simulink library "inp"  (R2021b)
settings: Solver=VariableStepAuto  StartTime=0.0  StopTime=10.0  RelTol=1e-3
undefined symbols (not defined in the file): C_TASK_5MS_S, FALSE, KINP_AcoreReadyToSlp_flg_ovrdflg, KINP_AcoreReadyToSlp_flg_ovrdval, KINP_AllowMovThd_OTA_enum_ovrdflg, KINP_AllowMovThd_OTA_enum_ovrdval, KINP_APSAngleTarget_Deg_ovrdflg, KINP_APSAngleTarget_Deg_ovrdval, KINP_APSDecReq_mps2_ovrdflg, KINP_APSDecReq_mps2_ovrdval, KINP_APSDecReqA_flg_ovrdflg, KINP_APSDecReqA_flg_ovrdval, KINP_APSDFLL_cm_ovrdflg, KINP_APSDFLL_cm_ovrdval, KINP_APSDFLR_cm_ovrdflg, KINP_APSDFLR_cm_ovrdval, KINP_APSDRLL_cm_ovrdflg, KINP_APSDRLL_cm_ovrdval, KINP_APSDRLR_cm_ovrdflg, KINP_APSDRLR_cm_ovrdval, KINP_APSExitCondition_enum_ovrdflg, KINP_APSExitCondition_enum_ovrdval, KINP_APSHWVer_enum_ovrdflg, KINP_APSHWVer_enum_ovrdval, KINP_APSProgressPCT_pct_ovrdflg, KINP_APSProgressPCT_pct_ovrdval, KINP_APSPwrReq_enum_ovrdflg, KINP_APSPwrReq_enum_ovrdval, KINP_APSReq_enum_ovrdflg, KINP_APSReq_enum_ovrdval, KINP_APSRQDisplay_enum_ovrdflg, KINP_APSRQDisplay_enum_ovrdval, KINP_APSRqEPASCtrl_flg_ovrdflg, KINP_APSRqEPASCtrl_flg_ovrdval, KINP_APSShiftPosnReq_enum_ovrdval, KINP_APSShiftPosnReq_enum_ovrflg, KINP_APSSpeedCMD_kph_ovrdval, KINP_APSSpeedCMD_kph_ovrflg, KINP_APSStaSystem_enum_ovrdflg, KINP_APSStaSystem_enum_ovrdval, KINP_APSSWVer_enum_ovrdflg, KINP_APSSWVer_enum_ovrdval, KINP_APSVMCReqA_flg_ovrdval, KINP_APSVMCReqA_flg_ovrflg, KINP_APSVRqEPASCtrl_flg_ovrdflg, KINP_APSVRqEPASCtrl_flg_ovrdval, KINP_AuxBattVolmV_mV_ovrdflg, KINP_AuxBattVolmV_mV_ovrdval, KINP_CAASSta_enum_ovrdflg, KINP_CAASSta_enum_ovrdval, KINP_CAASVMCReqA_flg_ovrdval, KINP_CAASVMCReqA_flg_ovrflg, KINP_CAN1BusOff_flg_ovrdflg, KINP_CAN1BusOff_flg_ovrdval, KINP_CAN2BusOff_flg_ovrdflg, KINP_CAN2BusOff_flg_ovrdval, KINP_CAN3BusOff_flg_ovrdflg, KINP_CAN3BusOff_flg_ovrdval, KINP_CAN4BusOff_flg_ovrdflg, KINP_CAN4BusOff_flg_ovrdval ... (+152)
libraries: FVT_lib x1035, hcu_lib x1
(part 3 of 33)

== system inp/INP/TPMS ==
  BHAL_TPMS_outputs : Inport  OutDataTypeStr=Bus: BHAL_TPMS_outputs
  Bus Creator : BusCreator  Inputs=52  OutDataTypeStr=Bus: BINP_TPMS_outputs  NonVirtualBus=on
  Bus Selector : BusSelector  OutputSignals=VHAL_TPMSDataIn_flg,VHAL_TPMSID_raw,VHAL_TPMSPressure_raw,VHAL_TPMSTemp_raw,VHAL_TPMSSta_enum,VHAL_TPMSPressureMi_raw,VHAL_TPMSCRC_crc,VHAL_TPMSCRCCalc_crc,VHAL_TPMSFAT_flg,VHAL_TPMSBattLow_flg,VHAL_TPMSStorge_flg,VHAL_LFID_raw,VHAL_RFID_raw,VHAL_LRID_raw,VHAL_RRID_raw,VHAL_ChkStorge_flg,VHAL_ChkLFID_raw,VHAL_ChkRFID_raw,VHAL_ChkLRID_raw,VHAL_ChkRRID_raw,VHAL_FlashLFSensorFail_flg,VHAL_FlashRFSensorFail_flg,VHAL_FlashLRSensorFail_flg,VHAL_FlashRRSensorFail_flg,VHAL_FlashLFWheelPSW_raw8,VHAL_FlashRFWheelPSW_raw8,VHAL_FlashLRWheelPSW_raw8,VHAL_FlashRRWheelPSW_raw8,VHAL_FlashLFPindi_enum,VHAL_FlashRFPindi_enum,VHAL_FlashLRPindi_enum,VHAL_FlashRRPindi_enum,VHAL_FlashLFP20_raw8,VHAL_FlashRFP20_raw8,VHAL_FlashLRP20_raw8,VHAL_FlashRRP20_raw8,VHAL_FlashLFWheelPress_raw8,VHAL_FlashRFWheelPress_raw8,VHAL_FlashLRWheelPress_raw8,VHAL_FlashRRWheelPress_raw8,VHAL_FlashLFWheelTemp_C,VHAL_FlashRFWheelTemp_C,VHAL_FlashLRWheelTemp_C,VHAL_FlashRRWheelTemp_C,VHAL_FlashunlearnSfali_flg,VHAL_S1ID_raw,VHAL_S2ID_raw,VHAL_S3ID_raw,VHAL_S4ID_raw,VHAL_Prepresstemptrust_flg,VHAL_TPMSSensorIDRegSta_enum,VHAL_TPMSTrigger_flg
  Data Type Conversion{,8..10,15,26,28,45..48,55} (12 alike) : DataTypeConversion  OutDataTypeStr=boolean
  Data Type Conversion{1,11..14,16..19,22..25} (13 alike) : DataTypeConversion  OutDataTypeStr=uint32
  Data Type Conversion{2..7,20..21,27,32,34..35,37..44,49..54,56} (27 alike) : DataTypeConversion  OutDataTypeStr=uint8
  Subsystem : Subsystem
  Subsystem1 : Subsystem
  Subsystem10 : Subsystem
  Subsystem11 : Subsystem
  Subsystem12 : Subsystem
  Subsystem13 : Subsystem
  Subsystem14 : Subsystem
  Subsystem2 : Subsystem
  Subsystem3 : Subsystem
  Subsystem4 : Subsystem
  Subsystem5 : Subsystem
  Subsystem6 : Subsystem
  Subsystem7 : Subsystem
  Subsystem8 : Subsystem
  Subsystem9 : Subsystem
  BINP_TPMS_outputs : Outport  OutDataTypeStr=Bus: BINP_TPMS_outputs
  wires:
  Bus Selector/49 -> Data Type Conversion25/1  "<VHAL_S4ID_raw>"
  Bus Selector/48 -> Data Type Conversion24/1  "<VHAL_S3ID_raw>"
  Bus Selector/47 -> Data Type Conversion23/1  "<VHAL_S2ID_raw>"
  Bus Selector/46 -> Data Type Conversion22/1  "<VHAL_S1ID_raw>"
  Data Type Conversion25/1 -> Bus Creator/49  "VINP_S4ID_raw"
  Data Type Conversion24/1 -> Bus Creator/48  "VINP_S3ID_raw"
  Data Type Conversion23/1 -> Bus Creator/47  "VINP_S2ID_raw"
  Data Type Conversion22/1 -> Bus Creator/46  "VINP_S1ID_raw"
  Data Type Conversion21/1 -> Bus Creator/44  "VINP_FlashRRWheelTemp_C"
  Data Type Conversion20/1 -> Bus Creator/43  "VINP_FlashLRWheelTemp_C"
  Bus Selector/44 -> Data Type Conversion21/1  "<VHAL_FlashRRWheelTemp_C>"
  Bus Selector/43 -> Data Type Conversion20/1  "<VHAL_FlashLRWheelTemp_C>"
  Data Type Conversion55/1 -> Bus Creator/45  "VINP_FlashunlearnSfali_flg"
  Bus Selector/45 -> Data Type Conversion55/1  "<VHAL_FlashunlearnSfali_flg>"
  Data Type Conversion44/1 -> Bus Creator/42  "VINP_FlashRFWheelTemp_C"
  Bus Selector/42 -> Data Type Conversion44/1  "<VHAL_FlashRFWheelTemp_C>"
  Data Type Conversion43/1 -> Bus Creator/41  "VINP_FlashLFWheelTemp_C"
  Bus Selector/41 -> Data Type Conversion43/1  "<VHAL_FlashLFWheelTemp_C>"
  Data Type Conversion54/1 -> Bus Creator/40  "VINP_FlashRRWheelPress_raw8"
  Data Type Conversion42/1 -> Bus Creator/39  "VINP_FlashLRWheelPress_raw8"
  Bus Selector/40 -> Data Type Conversion54/1  "<VHAL_FlashRRWheelPress_raw8>"
  Bus Selector/39 -> Data Type Conversion42/1  "<VHAL_FlashLRWheelPress_raw8>"
  Data Type Conversion34/1 -> Bus Creator/38  "VINP_FlashRFWheelPress_raw8"
  Bus Selector/38 -> Data Type Conversion34/1  "<VHAL_FlashRFWheelPress_raw8>"
  Data Type Conversion56/1 -> Bus Creator/37  "VINP_FlashLFWheelPress_raw8"
  Bus Selector/37 -> Data Type Conversion56/1  "<VHAL_FlashLFWheelPress_raw8>"
  Data Type Conversion41/1 -> Bus Creator/36  "VINP_FlashRRP20_raw8"
  Bus Selector/36 -> Data Type Conversion41/1  "<VHAL_FlashRRP20_raw8>"
  Data Type Conversion39/1 -> Bus Creator/35  "VINP_FlashLRP20_raw8"
  Bus Selector/35 -> Data Type Conversion39/1  "<VHAL_FlashLRP20_raw8>"
  Data Type Conversion38/1 -> Bus Creator/34  "VINP_FlashRFP20_raw8"
  Bus Selector/34 -> Data Type Conversion38/1  "<VHAL_FlashRFP20_raw8>"
  Data Type Conversion40/1 -> Bus Creator/33  "VINP_FlashLFP20_raw8"
  Bus Selector/33 -> Data Type Conversion40/1  "<VHAL_FlashLFP20_raw8>"
  Data Type Conversion37/1 -> Bus Creator/32  "VINP_FlashRRPindi_enum"
  Bus Selector/32 -> Data Type Conversion37/1  "<VHAL_FlashRRPindi_enum>"
  Data Type Conversion35/1 -> Bus Creator/31  "VINP_FlashLRPindi_enum"
  Bus Selector/31 -> Data Type Conversion35/1  "<VHAL_FlashLRPindi_enum>"
  Data Type Conversion53/1 -> Bus Creator/30  "VINP_FlashRFPindi_enum"
  Bus Selector/30 -> Data Type Conversion53/1  "<VHAL_FlashRFPindi_enum>"
  Data Type Conversion32/1 -> Bus Creator/29  "VINP_FlashLFPindi_enum"
  Bus Selector/29 -> Data Type Conversion32/1  "<VHAL_FlashLFPindi_enum>"
  Data Type Conversion52/1 -> Bus Creator/28  "VINP_FlashRRWheelPSW_raw8"
  Bus Selector/28 -> Data Type Conversion52/1  "<VHAL_FlashRRWheelPSW_raw8>"
  Data Type Conversion50/1 -> Bus Creator/27  "VINP_FlashLRWheelPSW_raw8"
  Bus Selector/27 -> Data Type Conversion50/1  "<VHAL_FlashLRWheelPSW_raw8>"
  Data Type Conversion49/1 -> Bus Creator/26  "VINP_FlashRFWheelPSW_raw8"
  Bus Selector/26 -> Data Type Conversion49/1  "<VHAL_FlashRFWheelPSW_raw8>"
  Data Type Conversion51/1 -> Bus Creator/25  "VINP_FlashLFWheelPSW_raw8"
  Bus Selector/25 -> Data Type Conversion51/1  "<VHAL_FlashLFWheelPSW_raw8>"
  Data Type Conversion48/1 -> Bus Creator/24  "VINP_FlashRRSensorFail_flg"
  Bus Selector/24 -> Data Type Conversion48/1  "<VHAL_FlashRRSensorFail_flg>"
  Data Type Conversion47/1 -> Bus Creator/23  "VINP_FlashLRSensorFail_flg"
  Bus Selector/23 -> Data Type Conversion47/1  "<VHAL_FlashLRSensorFail_flg>"
  Data Type Conversion46/1 -> Bus Creator/22  "VINP_FlashRFSensorFail_flg"
  Bus Selector/22 -> Data Type Conversion46/1  "<VHAL_FlashRFSensorFail_flg>"
  Data Type Conversion45/1 -> Bus Creator/21  "VINP_FlashLFSensorFail_flg"
  Bus Selector/21 -> Data Type Conversion45/1  "<VHAL_FlashLFSensorFail_flg>"
  Data Type Conversion19/1 -> Bus Creator/20  "VINP_ChkRRID_raw"
  Data Type Conversion18/1 -> Bus Creator/19  "VINP_ChkLRID_raw"
  Data Type Conversion17/1 -> Bus Creator/18  "VINP_ChkRFID_raw"
  Data Type Conversion16/1 -> Bus Creator/17  "VINP_ChkLFID_raw"
  Data Type Conversion15/1 -> Bus Creator/16  "VINP_ChkStorge_flg"
  Bus Selector/20 -> Data Type Conversion19/1  "<VHAL_ChkRRID_raw>"
  Bus Selector/19 -> Data Type Conversion18/1  "<VHAL_ChkLRID_raw>"
  Bus Selector/18 -> Data Type Conversion17/1  "<VHAL_ChkRFID_raw>"
  Bus Selector/17 -> Data Type Conversion16/1  "<VHAL_ChkLFID_raw>"
  Bus Selector/16 -> Data Type Conversion15/1  "<VHAL_ChkStorge_flg>"
  Data Type Conversion14/1 -> Bus Creator/15  "VINP_RRID_raw"
  Data Type Conversion13/1 -> Bus Creator/14  "VINP_LRID_raw"
  Data Type Conversion12/1 -> Bus Creator/13  "VINP_RFID_raw"
  Data Type Conversion11/1 -> Bus Creator/12  "VINP_LFID_raw"
  Subsystem14/1(Out1) -> Data Type Conversion14/1
  Subsystem13/1(Out1) -> Data Type Conversion13/1
  Subsystem12/1(Out1) -> Data Type Conversion12/1
  Subsystem11/1(Out1) -> Data Type Conversion11/1
  Bus Selector/15 -> Subsystem14/1(In1)  "<VHAL_RRID_raw>"
  Bus Selector/14 -> Subsystem13/1(In1)  "<VHAL_LRID_raw>"
  Bus Selector/13 -> Subsystem12/1(In1)  "<VHAL_RFID_raw>"
  Bus Selector/12 -> Subsystem11/1(In1)  "<VHAL_LFID_raw>"
  Data Type Conversion10/1 -> Bus Creator/11  "VINP_TPMSStorge_flg"
  Subsystem10/1(Out1) -> Data Type Conversion10/1
  Bus Selector/11 -> Subsystem10/1(In1)  "<VHAL_TPMSStorge_flg>"
  Subsystem9/1(Out1) -> Data Type Conversion9/1
  Subsystem8/1(Out1) -> Data Type Conversion8/1
  Bus Selector/10 -> Subsystem9/1(In1)  "<VHAL_TPMSBattLow_flg>"
  Bus Selector/9 -> Subsystem8/1(In1)  "<VHAL_TPMSFAT_flg>"
  Data Type Conversion9/1 -> Bus Creator/10  "VINP_TPMSBattLow_flg"
  Data Type Conversion8/1 -> Bus Creator/9  "VINP_TPMSFAT_flg"
  Bus Creator/1 -> BINP_TPMS_outputs/1
  Data Type Conversion7/1 -> Bus Creator/8  "VINP_TPMSCRCCalc_crc"
  Data Type Conversion6/1 -> Bus Creator/7  "VINP_TPMSCRC_crc"
  Data Type Conversion5/1 -> Bus Creator/6  "VINP_TPMSPressureMi_raw"
  Data Type Conversion4/1 -> Bus Creator/5  "VINP_TPMSSta_enum"
  Data Type Conversion3/1 -> Bus Creator/4  "VINP_TPMSTemp_raw"
  Data Type Conversion2/1 -> Bus Creator/3  "VINP_TPMSPressure_raw"
  Data Type Conversion1/1 -> Bus Creator/2  "VINP_TPMSID_raw"
  Data Type Conversion/1 -> Bus Creator/1  "VINP_TPMSDataIn_flg"
  Subsystem7/1(Out1) -> Data Type Conversion7/1
  Subsystem6/1(Out1) -> Data Type Conversion6/1
  Subsystem5/1(Out1) -> Data Type Conversion5/1
  Subsystem4/1(Out1) -> Data Type Conversion4/1
  Subsystem3/1(Out1) -> Data Type Conversion3/1
  Subsystem2/1(Out1) -> Data Type Conversion2/1
  Subsystem1/1(Out1) -> Data Type Conversion1/1
  Subsystem/1(Out1) -> Data Type Conversion/1
  Bus Selector/8 -> Subsystem7/1(In1)  "<VHAL_TPMSCRCCalc_crc>"
  Bus Selector/7 -> Subsystem6/1(In1)  "<VHAL_TPMSCRC_crc>"
  Bus Selector/6 -> Subsystem5/1(In1)  "<VHAL_TPMSPressureMi_raw>"
  Bus Selector/5 -> Subsystem4/1(In1)  "<VHAL_TPMSSta_enum>"
  Bus Selector/4 -> Subsystem3/1(In1)  "<VHAL_TPMSTemp_raw>"
  Bus Selector/3 -> Subsystem2/1(In1)  "<VHAL_TPMSPressure_raw>"
  Bus Selector/2 -> Subsystem1/1(In1)  "<VHAL_TPMSID_raw>"
  Bus Selector/1 -> Subsystem/1(In1)  "<VHAL_TPMSDataIn_flg>"
  BHAL_TPMS_outputs/1 -> Bus Selector/1
  Bus Selector/50 -> Data Type Conversion26/1  "<VHAL_Prepresstemptrust_flg>"
  Data Type Conversion26/1 -> Bus Creator/50  "VINP_Prepresstemptrust_flg"
  Bus Selector/51 -> Data Type Conversion27/1  "<VHAL_TPMSSensorIDRegSta_enum>"
  Data Type Conversion27/1 -> Bus Creator/51  "VINP_TPMSSensorIDRegSta_enum"
  Bus Selector/52 -> Data Type Conversion28/1  "<VHAL_TPMSTrigger_flg>"
  Data Type Conversion28/1 -> Bus Creator/52  "VINP_TPMSTrigger_flg"

== system inp/INP/APM/Subsystem ==
  In1 : Inport
  Constant : Constant  Value=KINP_PASDRMR_cm_ovrdval
  Constant1 : Constant  Value=KINP_PASDRMR_cm_ovrdflg
  Switch : Switch  Criteria=u2 ~= 0
  Out1 : Outport
  wires:
  Switch/1 -> Out1/1
  In1/1 -> Switch/3
  Constant/1 -> Switch/1
  Constant1/1 -> Switch/2

== system inp/INP/APM/Subsystem1 ==
  In1 : Inport
  Constant : Constant  Value=KINP_PASDRML_cm_ovrdval
  Constant1 : Constant  Value=KINP_PASDRML_cm_ovrdflg
  Switch : Switch  Criteria=u2 ~= 0
  Out1 : Outport
  wires:
  Constant1/1 -> Switch/2
  Constant/1 -> Switch/1
  In1/1 -> Switch/3
  Switch/1 -> Out1/1

== system inp/INP/APM/Subsystem10 ==
  In1 : Inport
  Constant : Constant  Value=KINP_APSDFLR_cm_ovrdval
  Constant1 : Constant  Value=KINP_APSDFLR_cm_ovrdflg
  Switch : Switch  Criteria=u2 ~= 0
  Out1 : Outport
  wires:
  Switch/1 -> Out1/1
  In1/1 -> Switch/3
  Constant/1 -> Switch/1
  Constant1/1 -> Switch/2

== system inp/INP/APM/Subsystem11 ==
  In1 : Inport
  Constant : Constant  Value=KINP_APSDFLL_cm_ovrdval
  Constant1 : Constant  Value=KINP_APSDFLL_cm_ovrdflg
  Switch : Switch  Criteria=u2 ~= 0
  Out1 : Outport
  wires:
  Constant1/1 -> Switch/2
  Constant/1 -> Switch/1
  In1/1 -> Switch/3
  Switch/1 -> Out1/1

== system inp/INP/APM/Subsystem12 ==
  In1 : Inport
  Constant : Constant  Value=KINP_PASAFCL_enum_ovrdval
  Constant1 : Constant  Value=KINP_PASAFCL_enum_ovrdflg
  Switch : Switch  Criteria=u2 ~= 0
  Out1 : Outport
  wires:
  Switch/1 -> Out1/1
  In1/1 -> Switch/3
  Constant/1 -> Switch/1
  Constant1/1 -> Switch/2

== system inp/INP/APM/Subsystem13 ==
  In1 : Inport
  Constant : Constant  Value=KINP_PASARMR_enum_ovrdval
  Constant1 : Constant  Value=KINP_PASARMR_enum_ovrdflg
  Switch : Switch  Criteria=u2 ~= 0
  Out1 : Outport
  wires:
  Constant1/1 -> Switch/2
  Constant/1 -> Switch/1
  In1/1 -> Switch/3
  Switch/1 -> Out1/1

== system inp/INP/APM/Subsystem14 ==
  In1 : Inport
  Constant : Constant  Value=KINP_PASARML_enum_ovrdval
  Constant1 : Constant  Value=KINP_PASARML_enum_ovrdflg
  Switch : Switch  Criteria=u2 ~= 0
  Out1 : Outport
  wires:
  Switch/1 -> Out1/1
  In1/1 -> Switch/3
  Constant/1 -> Switch/1
  Constant1/1 -> Switch/2

== system inp/INP/APM/Subsystem15 ==
  In1 : Inport
  Constant : Constant  Value=KINP_PASARCR_enum_ovrdval
  Constant1 : Constant  Value=KINP_PASARCR_enum_ovrdflg
  Switch : Switch  Criteria=u2 ~= 0
  Out1 : Outport
  wires:
  Constant1/1 -> Switch/2
  Constant/1 -> Switch/1
  In1/1 -> Switch/3
  Switch/1 -> Out1/1

== system inp/INP/APM/Subsystem16 ==
  In1 : Inport
  Constant : Constant  Value=KINP_PASARCL_enum_ovrdval
  Constant1 : Constant  Value=KINP_PASARCL_enum_ovrdflg
  Switch : Switch  Criteria=u2 ~= 0
  Out1 : Outport
  wires:
  Switch/1 -> Out1/1
  In1/1 -> Switch/3
  Constant/1 -> Switch/1
  Constant1/1 -> Switch/2

== system inp/INP/APM/Subsystem17 ==
  In1 : Inport
  Constant : Constant  Value=KINP_PASAFMR_enum_ovrdval
  Constant1 : Constant  Value=KINP_PASAFMR_enum_ovrdflg
  Switch : Switch  Criteria=u2 ~= 0
  Out1 : Outport
  wires:
  Constant1/1 -> Switch/2
  Constant/1 -> Switch/1
  In1/1 -> Switch/3
  Switch/1 -> Out1/1

== system inp/INP/APM/Subsystem18 ==
  In1 : Inport
  Constant : Constant  Value=KINP_PASAFML_enum_ovrdval
  Constant1 : Constant  Value=KINP_PASAFML_enum_ovrdflg
  Switch : Switch  Criteria=u2 ~= 0
  Out1 : Outport
  wires:
  Switch/1 -> Out1/1
  In1/1 -> Switch/3
  Constant/1 -> Switch/1
  Constant1/1 -> Switch/2

== system inp/INP/APM/Subsystem19 ==
  In1 : Inport
  Constant : Constant  Value=KINP_PASAFCR_enum_ovrdval
  Constant1 : Constant  Value=KINP_PASAFCR_enum_ovrdflg
  Switch : Switch  Criteria=u2 ~= 0
  Out1 : Outport
  wires:
  Constant1/1 -> Switch/2
  Constant/1 -> Switch/1
  In1/1 -> Switch/3
  Switch/1 -> Out1/1

== system inp/INP/APM/Subsystem2 ==
  In1 : Inport
  Constant : Constant  Value=KINP_PASDRCR_cm_ovrdval
  Constant1 : Constant  Value=KINP_PASDRCR_cm_ovrdflg
  Switch : Switch  Criteria=u2 ~= 0
  Out1 : Outport
  wires:
  Constant1/1 -> Switch/2
  Constant/1 -> Switch/1
  In1/1 -> Switch/3
  Switch/1 -> Out1/1

== system inp/INP/APM/Subsystem20 ==
  In1 : Inport
  Constant : Constant  Value=KINP_USSStaRMR_flg_ovrdval
  Constant1 : Constant  Value=KINP_USSStaRMR_flg_ovrdflg
  Switch : Switch  Criteria=u2 ~= 0
  Out1 : Outport
  wires:
  Switch/1 -> Out1/1
  In1/1 -> Switch/3
  Constant/1 -> Switch/1
  Constant1/1 -> Switch/2

== system inp/INP/APM/Subsystem21 ==
  In1 : Inport
  Constant : Constant  Value=KINP_USSStaRML_flg_ovrdval
  Constant1 : Constant  Value=KINP_USSStaRML_flg_ovrdflg
  Switch : Switch  Criteria=u2 ~= 0
  Out1 : Outport
  wires:
  Constant1/1 -> Switch/2
  Constant/1 -> Switch/1
  In1/1 -> Switch/3
  Switch/1 -> Out1/1

== system inp/INP/APM/Subsystem22 ==
  In1 : Inport
  Constant : Constant  Value=KINP_USSStaRLR_flg_ovrdval
  Constant1 : Constant  Value=KINP_USSStaRLR_flg_ovrdflg
  Switch : Switch  Criteria=u2 ~= 0
  Out1 : Outport
  wires:
  Switch/1 -> Out1/1
  In1/1 -> Switch/3
  Constant/1 -> Switch/1
  Constant1/1 -> Switch/2

== system inp/INP/APM/Subsystem23 ==
  In1 : Inport
  Constant : Constant  Value=KINP_USSStaRLL_flg_ovrdval
  Constant1 : Constant  Value=KINP_USSStaRLL_flg_ovrdflg
  Switch : Switch  Criteria=u2 ~= 0
  Out1 : Outport
  wires:
  Constant1/1 -> Switch/2
  Constant/1 -> Switch/1
  In1/1 -> Switch/3
  Switch/1 -> Out1/1

== system inp/INP/APM/Subsystem24 ==
  In1 : Inport
  Constant : Constant  Value=KINP_USSStaRCR_flg_ovrdval
  Constant1 : Constant  Value=KINP_USSStaRCR_flg_ovrdflg
  Switch : Switch  Criteria=u2 ~= 0
  Out1 : Outport
  wires:
  Switch/1 -> Out1/1
  In1/1 -> Switch/3
  Constant/1 -> Switch/1
  Constant1/1 -> Switch/2

== system inp/INP/APM/Subsystem25 ==
  In1 : Inport
  Constant : Constant  Value=KINP_USSStaRCL_flg_ovrdval
  Constant1 : Constant  Value=KINP_USSStaRCL_flg_ovrdflg
  Switch : Switch  Criteria=u2 ~= 0
  Out1 : Outport
  wires:
  Constant1/1 -> Switch/2
  Constant/1 -> Switch/1
  In1/1 -> Switch/3
  Switch/1 -> Out1/1

== system inp/INP/APM/Subsystem26 ==
  In1 : Inport
  Constant : Constant  Value=KINP_USSStaFMR_flg_ovrdval
  Constant1 : Constant  Value=KINP_USSStaFMR_flg_ovrdflg
  Switch : Switch  Criteria=u2 ~= 0
  Out1 : Outport
  wires:
  Switch/1 -> Out1/1
  In1/1 -> Switch/3
  Constant/1 -> Switch/1
  Constant1/1 -> Switch/2

== system inp/INP/APM/Subsystem27 ==
  In1 : Inport
  Constant : Constant  Value=KINP_USSStaFML_flg_ovrdval
  Constant1 : Constant  Value=KINP_USSStaFML_flg_ovrdflg
  Switch : Switch  Criteria=u2 ~= 0
  Out1 : Outport
  wires:
  Constant1/1 -> Switch/2
  Constant/1 -> Switch/1
  In1/1 -> Switch/3
  Switch/1 -> Out1/1

== system inp/INP/APM/Subsystem28 ==
  In1 : Inport
  Constant : Constant  Value=KINP_USSStaFLR_flg_ovrdval
  Constant1 : Constant  Value=KINP_USSStaFLR_flg_ovrdflg
  Switch : Switch  Criteria=u2 ~= 0
  Out1 : Outport
  wires:
  Switch/1 -> Out1/1
  In1/1 -> Switch/3
  Constant/1 -> Switch/1
  Constant1/1 -> Switch/2

== system inp/INP/APM/Subsystem29 ==
  In1 : Inport
  Constant : Constant  Value=KINP_USSStaFLL_flg_ovrdval
  Constant1 : Constant  Value=KINP_USSStaFLL_flg_ovrdflg
  Switch : Switch  Criteria=u2 ~= 0
  Out1 : Outport
  wires:
  Constant1/1 -> Switch/2
  Constant/1 -> Switch/1
  In1/1 -> Switch/3
  Switch/1 -> Out1/1

== system inp/INP/APM/Subsystem3 ==
  In1 : Inport
  Constant : Constant  Value=KINP_PASDRCL_cm_ovrdval
  Constant1 : Constant  Value=KINP_PASDRCL_cm_ovrdflg
  Switch : Switch  Criteria=u2 ~= 0
  Out1 : Outport
  wires:
  Constant1/1 -> Switch/2
  Constant/1 -> Switch/1
  In1/1 -> Switch/3
  Switch/1 -> Out1/1

== system inp/INP/APM/Subsystem30 ==
  In1 : Inport
  Constant : Constant  Value=KINP_USSStaFCR_flg_ovrdval
  Constant1 : Constant  Value=KINP_USSStaFCR_flg_ovrdflg
  Switch : Switch  Criteria=u2 ~= 0
  Out1 : Outport
  wires:
  Switch/1 -> Out1/1
  In1/1 -> Switch/3
  Constant/1 -> Switch/1
  Constant1/1 -> Switch/2

== system inp/INP/APM/Subsystem31 ==
  In1 : Inport
  Constant : Constant  Value=KINP_USSStaFCL_flg_ovrdval
  Constant1 : Constant  Value=KINP_USSStaFCL_flg_ovrdflg
  Switch : Switch  Criteria=u2 ~= 0
  Out1 : Outport
  wires:
  Constant1/1 -> Switch/2
  Constant/1 -> Switch/1
  In1/1 -> Switch/3
  Switch/1 -> Out1/1

== system inp/INP/APM/Subsystem32 ==
  In1 : Inport
  Constant : Constant  Value=KINP_Chime_enum_ovrdval
  Constant1 : Constant  Value=KINP_Chime_enum_ovrdflg
  Switch : Switch  Criteria=u2 ~= 0
  Out1 : Outport
  wires:
  Switch/1 -> Out1/1
  In1/1 -> Switch/3
  Constant/1 -> Switch/1
  Constant1/1 -> Switch/2

== system inp/INP/APM/Subsystem33 ==
  In1 : Inport
  Constant : Constant  Value=KINP_SNSRLayout_enum_ovrdval
  Constant1 : Constant  Value=KINP_SNSRLayout_enum_ovrdflg
  Switch : Switch  Criteria=u2 ~= 0
  Out1 : Outport
  wires:
  Constant1/1 -> Switch/2
  Constant/1 -> Switch/1
  In1/1 -> Switch/3
  Switch/1 -> Out1/1

== system inp/INP/APM/Subsystem34 ==
  In1 : Inport
  Constant : Constant  Value=KINP_StaFSya_flg_ovrdval
  Constant1 : Constant  Value=KINP_StaFSya_flg_ovrdflg
  Switch : Switch  Criteria=u2 ~= 0
  Out1 : Outport
  wires:
  Switch/1 -> Out1/1
  In1/1 -> Switch/3
  Constant/1 -> Switch/1
  Constant1/1 -> Switch/2

== system inp/INP/APM/Subsystem35 ==
  In1 : Inport
  Constant : Constant  Value=KINP_ModOperation_enum_ovrdval
  Constant1 : Constant  Value=KINP_ModOperation_enum_ovrdflg
  Switch : Switch  Criteria=u2 ~= 0
  Out1 : Outport
  wires:
  Constant1/1 -> Switch/2
  Constant/1 -> Switch/1
  In1/1 -> Switch/3
  Switch/1 -> Out1/1

== system inp/INP/APM/Subsystem36 ==
  In1 : Inport
  Constant : Constant  Value=KINP_APSVMCReqA_flg_ovrflg
  Constant1 : Constant  Value=KINP_APSVMCReqA_flg_ovrdval
  Switch : Switch  Criteria=u2 ~= 0
  Out1 : Outport
  wires:
  Constant/1 -> Switch/2
  Constant1/1 -> Switch/1
  In1/1 -> Switch/3
  Switch/1 -> Out1/1

== system inp/INP/APM/Subsystem37 ==
  In1 : Inport
  Constant : Constant  Value=KINP_APSShiftPosnReq_enum_ovrflg
  Constant1 : Constant  Value=KINP_APSShiftPosnReq_enum_ovrdval
  Switch : Switch  Criteria=u2 ~= 0
  Out1 : Outport
  wires:
  Switch/1 -> Out1/1
  In1/1 -> Switch/3
  Constant1/1 -> Switch/1
  Constant/1 -> Switch/2

== system inp/INP/APM/Subsystem38 ==
  In1 : Inport
  Constant : Constant  Value=KINP_APSSpeedCMD_kph_ovrflg
  Constant1 : Constant  Value=KINP_APSSpeedCMD_kph_ovrdval
  Switch : Switch  Criteria=u2 ~= 0
  Out1 : Outport
  wires:
  Constant/1 -> Switch/2
  Constant1/1 -> Switch/1
  In1/1 -> Switch/3
  Switch/1 -> Out1/1

== system inp/INP/APM/Subsystem39 ==
  In1 : Inport
  Constant : Constant  Value=KINP_CAASVMCReqA_flg_ovrflg
  Constant1 : Constant  Value=KINP_CAASVMCReqA_flg_ovrdval
  Switch : Switch  Criteria=u2 ~= 0
  Out1 : Outport
  wires:
  Switch/1 -> Out1/1
  In1/1 -> Switch/3
  Constant1/1 -> Switch/1
  Constant/1 -> Switch/2

== system inp/INP/APM/Subsystem4 ==
  In1 : Inport
  Constant : Constant  Value=KINP_PASDFMR_cm_ovrdval
  Constant1 : Constant  Value=KINP_PASDFMR_cm_ovrdflg
  Switch : Switch  Criteria=u2 ~= 0
  Out1 : Outport
  wires:
  Switch/1 -> Out1/1
  In1/1 -> Switch/3
  Constant/1 -> Switch/1
  Constant1/1 -> Switch/2

== system inp/INP/APM/Subsystem40 ==
  In1 : Inport
  Constant : Constant  Value=KINP_APSProgressPCT_pct_ovrdval
  Constant1 : Constant  Value=KINP_APSProgressPCT_pct_ovrdflg
  Switch : Switch  Criteria=u2 ~= 0
  Out1 : Outport
  wires:
  Switch/1 -> Out1/1
  In1/1 -> Switch/3
  Constant/1 -> Switch/1
  Constant1/1 -> Switch/2

== system inp/INP/APM/Subsystem41 ==
  In1 : Inport
  Constant : Constant  Value=KINP_APSRQDisplay_enum_ovrdval
  Constant1 : Constant  Value=KINP_APSRQDisplay_enum_ovrdflg
  Switch : Switch  Criteria=u2 ~= 0
  Out1 : Outport
  wires:
  Switch/1 -> Out1/1
  In1/1 -> Switch/3
  Constant/1 -> Switch/1
  Constant1/1 -> Switch/2

== system inp/INP/APM/Subsystem42 ==
  In1 : Inport
  Constant : Constant  Value=KINP_APSSWVer_enum_ovrdval
  Constant1 : Constant  Value=KINP_APSSWVer_enum_ovrdflg
  Switch : Switch  Criteria=u2 ~= 0
  Out1 : Outport
  wires:
  Switch/1 -> Out1/1
  In1/1 -> Switch/3
  Constant/1 -> Switch/1
  Constant1/1 -> Switch/2

== system inp/INP/APM/Subsystem43 ==
  In1 : Inport
  Constant : Constant  Value=KINP_APSHWVer_enum_ovrdval
  Constant1 : Constant  Value=KINP_APSHWVer_enum_ovrdflg
  Switch : Switch  Criteria=u2 ~= 0
  Out1 : Outport
  wires:
  Switch/1 -> Out1/1
  In1/1 -> Switch/3
  Constant/1 -> Switch/1
  Constant1/1 -> Switch/2

== system inp/INP/APM/Subsystem44 ==
  In1 : Inport
  Constant : Constant  Value=KINP_APSExitCondition_enum_ovrdval
  Constant1 : Constant  Value=KINP_APSExitCondition_enum_ovrdflg
  Switch : Switch  Criteria=u2 ~= 0
  Out1 : Outport
  wires:
  Switch/1 -> Out1/1
  In1/1 -> Switch/3
  Constant/1 -> Switch/1
  Constant1/1 -> Switch/2

== system inp/INP/APM/Subsystem45 ==
  In1 : Inport
  Constant : Constant  Value=KINP_APSAngleTarget_Deg_ovrdval
  Constant1 : Constant  Value=KINP_APSAngleTarget_Deg_ovrdflg
  Switch : Switch  Criteria=u2 ~= 0
  Out1 : Outport
  wires:
  Switch/1 -> Out1/1
  In1/1 -> Switch/3
  Constant/1 -> Switch/1
  Constant1/1 -> Switch/2

== system inp/INP/APM/Subsystem46 ==
  In1 : Inport
  Constant : Constant  Value=KINP_APSStaSystem_enum_ovrdval
  Constant1 : Constant  Value=KINP_APSStaSystem_enum_ovrdflg
  Switch : Switch  Criteria=u2 ~= 0
  Out1 : Outport
  wires:
  Switch/1 -> Out1/1
  In1/1 -> Switch/3
  Constant/1 -> Switch/1
  Constant1/1 -> Switch/2

== system inp/INP/APM/Subsystem47 ==
  In1 : Inport
  Constant : Constant  Value=KINP_APSVRqEPASCtrl_flg_ovrdval
  Constant1 : Constant  Value=KINP_APSVRqEPASCtrl_flg_ovrdflg
  Switch : Switch  Criteria=u2 ~= 0
  Out1 : Outport
  wires:
  Constant1/1 -> Switch/2
  Constant/1 -> Switch/1
  In1/1 -> Switch/3
  Switch/1 -> Out1/1

== system inp/INP/APM/Subsystem48 ==
  In1 : Inport
  Constant : Constant  Value=KINP_APSRqEPASCtrl_flg_ovrdval
  Constant1 : Constant  Value=KINP_APSRqEPASCtrl_flg_ovrdflg
  Switch : Switch  Criteria=u2 ~= 0
  Out1 : Outport
  wires:
  Switch/1 -> Out1/1
  In1/1 -> Switch/3
  Constant/1 -> Switch/1
  Constant1/1 -> Switch/2

== system inp/INP/APM/Subsystem49 ==
  In1 : Inport
  Constant : Constant  Value=KINP_APSReq_enum_ovrdval
  Constant1 : Constant  Value=KINP_APSReq_enum_ovrdflg
  Switch : Switch  Criteria=u2 ~= 0
  Out1 : Outport
  wires:
  Constant1/1 -> Switch/2
  Constant/1 -> Switch/1
  In1/1 -> Switch/3
  Switch/1 -> Out1/1

== system inp/INP/APM/Subsystem5 ==
  In1 : Inport
  Constant : Constant  Value=KINP_PASDFML_cm_ovrdval
  Constant1 : Constant  Value=KINP_PASDFML_cm_ovrdflg
  Switch : Switch  Criteria=u2 ~= 0
  Out1 : Outport
  wires:
  Constant1/1 -> Switch/2
  Constant/1 -> Switch/1
  In1/1 -> Switch/3
  Switch/1 -> Out1/1

== system inp/INP/APM/Subsystem50 ==
  In1 : Inport
  Constant : Constant  Value=KINP_APSDecReq_mps2_ovrdval
  Constant1 : Constant  Value=KINP_APSDecReq_mps2_ovrdflg
  Switch : Switch  Criteria=u2 ~= 0
  Out1 : Outport
  wires:
  Constant1/1 -> Switch/2
  Constant/1 -> Switch/1
  In1/1 -> Switch/3
  Switch/1 -> Out1/1

== system inp/INP/APM/Subsystem51 ==
  In1 : Inport
  Constant : Constant  Value=KINP_APSDecReqA_flg_ovrdval
  Constant1 : Constant  Value=KINP_APSDecReqA_flg_ovrdflg
  Switch : Switch  Criteria=u2 ~= 0
  Out1 : Outport
  wires:
  Constant1/1 -> Switch/2
  Constant/1 -> Switch/1
  In1/1 -> Switch/3
  Switch/1 -> Out1/1

== system inp/INP/APM/Subsystem52 ==
  In1 : Inport
  Constant : Constant  Value=KINP_CAASSta_enum_ovrdval
  Constant1 : Constant  Value=KINP_CAASSta_enum_ovrdflg
  Switch : Switch  Criteria=u2 ~= 0
  Out1 : Outport
  wires:
  Constant1/1 -> Switch/2
  Constant/1 -> Switch/1
  In1/1 -> Switch/3
  Switch/1 -> Out1/1

== system inp/INP/APM/Subsystem53 ==
  In1 : Inport
  Constant : Constant  Value=KINP_APSPwrReq_enum_ovrdflg
  Constant1 : Constant  Value=KINP_APSPwrReq_enum_ovrdval
  Switch : Switch  Criteria=u2 ~= 0
  Out1 : Outport
  wires:
  Switch/1 -> Out1/1
  Constant1/1 -> Switch/1
  Constant/1 -> Switch/2
  In1/1 -> Switch/3

== system inp/INP/APM/Subsystem54 ==
  In1 : Inport
  Constant : Constant  Value=KINP_RAPSBCMLamp_enum_ovrdflg
  Constant1 : Constant  Value=KINP_RAPSBCMLamp_enum_ovrdval
  Switch : Switch  Criteria=u2 ~= 0
  Out1 : Outport
  wires:
  Constant/1 -> Switch/2
  Constant1/1 -> Switch/1
  In1/1 -> Switch/3
  Switch/1 -> Out1/1

== system inp/INP/APM/Subsystem55 ==
  In1 : Inport
  Constant : Constant  Value=KINP_RAPSBCMLockReq_flg_ovrdval
  Constant1 : Constant  Value=KINP_RAPSBCMLockReq_flg_ovrflg
  Switch : Switch  Criteria=u2 ~= 0
  Out1 : Outport
  wires:
  Switch/1 -> Out1/1
  Constant/1 -> Switch/1
  Constant1/1 -> Switch/2
  In1/1 -> Switch/3

== system inp/INP/APM/Subsystem56 ==
  In1 : Inport
  Constant : Constant  Value=KINP_RAPSErrLv1_flg_ovrflg
  Constant1 : Constant  Value=KINP_RAPSErrLv1_flg_ovrdval
  Switch : Switch  Criteria=u2 ~= 0
  Out1 : Outport
  wires:
  Switch/1 -> Out1/1
  Constant1/1 -> Switch/1
  Constant/1 -> Switch/2
  In1/1 -> Switch/3

== system inp/INP/APM/Subsystem57 ==
  In1 : Inport
  Constant : Constant  Value=KINP_RAPSErrWarnSta_enum_ovrdval
  Constant1 : Constant  Value=KINP_RAPSErrWarnSta_enum_ovrdflg
  Switch : Switch  Criteria=u2 ~= 0
  Out1 : Outport
  wires:
  Constant1/1 -> Switch/2
  Constant/1 -> Switch/1
  Switch/1 -> Out1/1
  In1/1 -> Switch/3

== system inp/INP/APM/Subsystem6 ==
  In1 : Inport
  Constant : Constant  Value=KINP_PASDFCR_cm_ovrdval
  Constant1 : Constant  Value=KINP_PASDFCR_cm_ovrdflg
  Switch : Switch  Criteria=u2 ~= 0
  Out1 : Outport
  wires:
  Switch/1 -> Out1/1
  In1/1 -> Switch/3
  Constant/1 -> Switch/1
  Constant1/1 -> Switch/2

== system inp/INP/APM/Subsystem7 ==
  In1 : Inport
  Constant : Constant  Value=KINP_PASDFCL_cm_ovrdval
  Constant1 : Constant  Value=KINP_PASDFCL_cm_ovrdflg
  Switch : Switch  Criteria=u2 ~= 0
  Out1 : Outport
  wires:
  Constant1/1 -> Switch/2
  Constant/1 -> Switch/1
  In1/1 -> Switch/3
  Switch/1 -> Out1/1

== system inp/INP/APM/Subsystem8 ==
  In1 : Inport
  Constant : Constant  Value=KINP_APSDRLR_cm_ovrdval
  Constant1 : Constant  Value=KINP_APSDRLR_cm_ovrdflg
  Switch : Switch  Criteria=u2 ~= 0
  Out1 : Outport
  wires:
  Switch/1 -> Out1/1
  In1/1 -> Switch/3
  Constant/1 -> Switch/1
  Constant1/1 -> Switch/2

== system inp/INP/APM/Subsystem9 ==
  In1 : Inport
  Constant : Constant  Value=KINP_APSDRLL_cm_ovrdval
  Constant1 : Constant  Value=KINP_APSDRLL_cm_ovrdflg
  Switch : Switch  Criteria=u2 ~= 0
  Out1 : Outport
  wires:
  Constant1/1 -> Switch/2
  Constant/1 -> Switch/1
  In1/1 -> Switch/3
  Switch/1 -> Out1/1

== system inp/INP/CAN1/CommunicationCheck ==
  BHAL_outputs : Inport
  CANMsgInvalidABM1 : FVT_lib/inp/CAN_Msg_Validity_Process_template  SystemSampleTime=-1  VariantActivationTime=update diagram  Latency=0  AutoFrameSizeCalculation=off
      link override ovrdflg: Value=KINP_CANMsgInvalidABM1_flg_ovrdflg
      link override ovrdval: Value=KINP_CANMsgInvalidABM1_flg_ovrdval
  CANMsgInvalidEPB1 : FVT_lib/inp/CAN_Msg_Validity_Process_template  SystemSampleTime=-1  VariantActivationTime=update diagram  Latency=0  AutoFrameSizeCalculation=off
      link override ovrdflg: Value=KINP_CANMsgInvalidEPB1_flg_ovrdflg
      link override ovrdval: Value=KINP_CANMsgInvalidEPB1_flg_ovrdval
  CANMsgInvalidEPS1 : FVT_lib/inp/CAN_Msg_Validity_Process_template  SystemSampleTime=-1  VariantActivationTime=update diagram  Latency=0  AutoFrameSizeCalculation=off
      link override ovrdflg: Value=KINP_CANMsgInvalidEPS1_flg_ovrdflg
      link override ovrdval: Value=KINP_CANMsgInvalidEPS1_flg_ovrdval
  CANMsgInvalidESC1 : FVT_lib/inp/CAN_Msg_Validity_Process_template  SystemSampleTime=-1  VariantActivationTime=update diagram  Latency=0  AutoFrameSizeCalculation=off
      link override ovrdflg: Value=KINP_CANMsgInvalidESC1_flg_ovrdflg
      link override ovrdval: Value=KINP_CANMsgInvalidESC1_flg_ovrdval
  CANMsgInvalidESC5 : FVT_lib/inp/CAN_Msg_Validity_Process_template  SystemSampleTime=-1  VariantActivationTime=update diagram  Latency=0  AutoFrameSizeCalculation=off
      link override ovrdflg: Value=KINP_CANMsgInvalidESC5_flg_ovrdflg
      link override ovrdval: Value=KINP_CANMsgInvalidESC5_flg_ovrdval
  CANMsgInvalideBST1 : FVT_lib/inp/CAN_Msg_Validity_Process_template  SystemSampleTime=-1  VariantActivationTime=update diagram  Latency=0  AutoFrameSizeCalculation=off
      link override ovrdflg: Value=KINP_CANMsgInvalideBST1_flg_ovrdflg
      link override ovrdval: Value=KINP_CANMsgInvalideBST1_flg_ovrdval
  bus_creator : BusCreator  Inputs=6
  bus_selector : BusSelector  OutputSignals=VHAL_CANMsgInvalidABM1_flg,VHAL_CANMsgInvalidEPB1_flg,VHAL_CANMsgInvalidEPS1_flg,VHAL_CANMsgInvalidESC1_flg,VHAL_CANMsgInvalidESC5_flg,VHAL_CANMsgInvalideBST1_flg
  not{1..6} (6 alike) : Logic  Operator=NOT  AllPortsSameDT=off  OutDataTypeStr=boolean
  inp_CanValid_bus : Outport
  wires:
  BHAL_outputs/1 -> [BHAL_outputs]
  bus_selector/1 -> CANMsgInvalidABM1/1  "<VHAL_CANMsgInvalidABM1_flg>"
  CANMsgInvalidABM1/1 -> not1/1
  not1/1 -> bus_creator/1  "VINP_CANMsgValidABM1_flg"
  bus_selector/2 -> CANMsgInvalidEPB1/1  "<VHAL_CANMsgInvalidEPB1_flg>"
  CANMsgInvalidEPB1/1 -> not2/1
  not2/1 -> bus_creator/2  "VINP_CANMsgValidEPB1_flg"
  bus_selector/3 -> CANMsgInvalidEPS1/1  "<VHAL_CANMsgInvalidEPS1_flg>"
  CANMsgInvalidEPS1/1 -> not3/1
  not3/1 -> bus_creator/3  "VINP_CANMsgValidEPS1_flg"
  bus_selector/4 -> CANMsgInvalidESC1/1  "<VHAL_CANMsgInvalidESC1_flg>"
  CANMsgInvalidESC1/1 -> not4/1
  not4/1 -> bus_creator/4  "VINP_CANMsgValidESC1_flg"
  bus_selector/5 -> CANMsgInvalidESC5/1  "<VHAL_CANMsgInvalidESC5_flg>"
  CANMsgInvalidESC5/1 -> not5/1
  not5/1 -> bus_creator/5  "VINP_CANMsgValidESC5_flg"
  bus_selector/6 -> CANMsgInvalideBST1/1  "<VHAL_CANMsgInvalideBST1_flg>"
  CANMsgInvalideBST1/1 -> not6/1
  not6/1 -> bus_creator/6  "VINP_CANMsgValideBST1_flg"
  [BHAL_outputs] -> bus_selector/1
  bus_creator/1 -> inp_CanValid_bus/1
